simulink model "liti4"  (Simulink 5.0)
settings: Solver=ode4  SolverMode=SingleTasking  StartTime=0.0  StopTime=10  FixedStep=0.01  RelTol=1e-3
libraries: cstblocks x2
settings Model: LastModifiedBy=Administrator

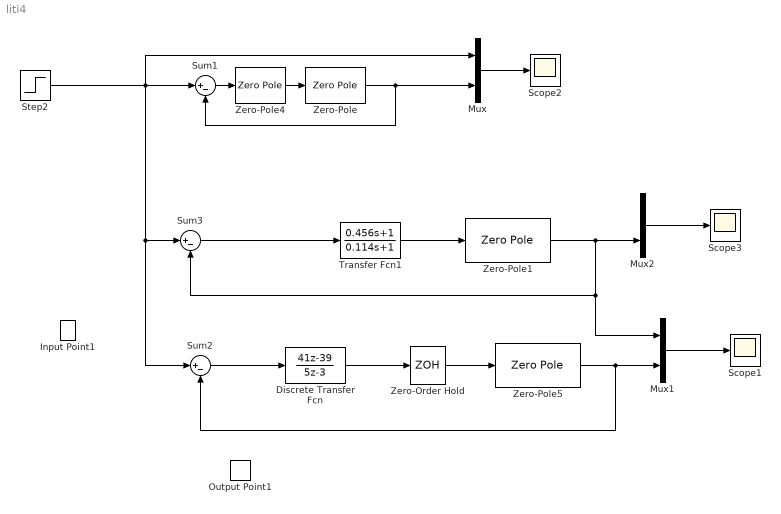
== system liti4 ==
  Discrete Transfer Fcn : DiscreteTransferFcn  Numerator=[41 -39]  Denominator=[5 -3]  SampleTime=0.01
  Input Point1 : cstblocks/Input Point
  Mux : Mux  Inputs=2
  Mux1 : Mux  Inputs=2
  Mux2 : Mux  Inputs=2
  Output Point1 : cstblocks/Output Point
  Scope1 : Scope
      settings: YMin=-3.5  YMax=1  MaxDataPoints=500000
  Scope2 : Scope
      settings: YMin=-3.5  YMax=1  MaxDataPoints=500000
  Scope3 : Scope
      settings: YMin=-3.5  YMax=1  SaveName=ScopeData2  MaxDataPoints=500000
  Step2 : Step  Time=0  SampleTime=0
  Sum1 : Sum  Inputs=|+-  SaturateOnIntegerOverflow=on
  Sum2 : Sum  Inputs=|+-  SaturateOnIntegerOverflow=on
  Sum3 : Sum  Inputs=|+-  SaturateOnIntegerOverflow=on
  Transfer Fcn1 : TransferFcn  Numerator=[0.456 1]  Denominator=[0.114 1]
  Zero-Order Hold : ZeroOrderHold  SampleTime=0.01
  Zero-Pole : ZeroPole  Zeros=[]  Poles=[0 -4]  Gain=[30*4]
  Zero-Pole1 : ZeroPole  Zeros=[]  Poles=[0 -1]  Gain=[10]
  Zero-Pole4 : ZeroPole  Zeros=[]  Poles=[-100]  Gain=[100]
  Zero-Pole5 : ZeroPole  Zeros=[]  Poles=[0 -1]  Gain=[10]
  wires:
  Sum1/1 -> Zero-Pole4/1
  Mux/1 -> Scope2/1
  Zero-Pole/1 -> Mux/2, Sum1/2
  Step2/1 -> Mux/1, Sum1/1, Sum2/1, Sum3/1
  Mux2/1 -> Scope3/1
  Zero-Pole1/1 -> Mux2/2, Mux1/1, Sum3/2
  Sum3/1 -> Transfer Fcn1/1
  Zero-Pole4/1 -> Zero-Pole/1
  Mux1/1 -> Scope1/1
  Zero-Pole5/1 -> Mux1/2, Sum2/2
  Discrete Transfer Fcn/1 -> Zero-Order Hold/1
  Sum2/1 -> Discrete Transfer Fcn/1
  Zero-Order Hold/1 -> Zero-Pole5/1
  Transfer Fcn1/1 -> Zero-Pole1/1
